simulink model "Model_TranslationEngine64"  (R2022b)
settings: Solver=FixedStepDiscrete  StartTime=0.0  StopTime=5  RelTol=1e-3  EnableMultiTasking=on
InitFcn:
  | % Initialize model
  | ModelSettings=BTConfig.GetModelSettings();
  | 
  | ModelSettings.Validate();
  | 
  | ModelInit;
  | 
  | 
  | % load library data
  | GainLibrary_data;
  | % Load saved values from partition process
  | CapturedConstMask.LoadMapFromFile(bdroot)
StartFcn:
  | % make sure all the simulated RTC requests are found
  | %RTC_SIM_OBJ.ValidateREQs();
undefined symbols (not defined in the file or in its folder): AA, BPLP, Column, NumHFRefBPF, NumHFRefLPF, NumMusicChannels, Row, VolumeMuteConfig
libraries: TuneVar x925, TOP x490, FeaturePath x111, CapturedConstLib x52
(part 27 of 34)

== system Model_TranslationEngine64/ModelPreAmp/DecRate/AudioPilot35/Audiopilot_3_5/NoiseEstimationVariant/RegularNoiseEstimation/HFNoiseEstimatorCoh/PostProcessing/HfImpulseRejection/MinSearch ==
  FlatnessHighIndex : Subsystem  mask(Talaria Trivial Tune TOP){TriggerInit=[-155 320 120 350], TopName=FlatnessHighIndex, TuneName=FlatnessHighIndex, DataTypeOut=single, MaskValue=Config.ImpRejFlatnessHighIndex, TunabilityNumber=1, MinValue=[], MaxValue=[], BankNumber=0, PreOverlay=false, PostOverlay=false, UseSameName=on}
      mask prompts: TriggerInit "Hidden: MoveFcn redraw"; TopName "Name:"; TuneName "Name of TuneVar:"; DataTypeOut "Data type:"; MaskValue "Default Value:"; TunabilityNumber "Tunability:"; MinValue "Min Value:"; MaxValue "Max Value:"; BankNumber "Target memory bank number:"; PreOverlay "Requires pre-overlay action:"; PostOverlay "Requires post-overlay action:"; UseSameName "Use same name for tune variable and TOP"
      mask help: The TuneTOP block encapsultes a Target Overlay Parameter, a Tune Variable, and a Trivial Translation between them.
      mask init:
      | [ok,activeTopPath,activeTunePath] = TuneTOP_Mask.Init(gcbh);
      settings: MoveFcn=TuneTOP_Mask.CB_TriggerInit(gcbh);
      mask Callback TriggerInit: TuneTOP_Mask.CB_TriggerInit(gcbh);
      mask TypeOptions TopName: TOP/TopName
      mask TypeOptions TuneName: Tune Variable/TuneName
      mask TypeOptions DataTypeOut: TOP/DataTypeOut
      mask TypeOptions MaskValue: Tune Variable/MaskValue
      mask TypeOptions TunabilityNumber: Tune Variable/TunabilityNumber
      mask Callback TunabilityNumber: TuneVarMask.CB_TunabilityNumber(gcbh);
      mask TypeOptions MinValue: Tune Variable/MinValue
      mask TypeOptions MaxValue: Tune Variable/MaxValue
      mask TypeOptions BankNumber: TOP/BankNumber
      mask TypeOptions PreOverlay: TOP/PreOverlay
      mask TypeOptions PostOverlay: TOP/PostOverlay
      mask Callback UseSameName: TuneTOP_Mask.CB_UseSameName(gcbh);
      mask DialogControl toolPanel Prompt: Tuning Tool Hints
      mask DialogControl DescriptionGroup Prompt: Description
      mask DialogControl EditDescription Prompt: Edit Description
      mask DialogControl EditDescription Callback: TuneTOP_Mask.CB_EditDescription(gcbh);
      mask DialogControl TunabilityText Prompt: Easy: Changes nearly every tuning.
      mask DialogControl AdvancedPanel Prompt: Advanced
      mask DialogControl ConvertToFullTranslation Prompt: Irreversible conversion to full translation
      mask DialogControl ConvertToFullTranslation Callback: TuneTOP_Mask.CB_ConvertToFullTranslation(gcbh);
      mask DialogControl ErrorContainer Prompt: Error Messages
      mask Display:
      | % retrieve icon definition
      | [path,w,h] = TuneTOP_Mask.Icon();
      | 
      | % retrieve the block's pixel size
      | pos = get(gcbh,'position');
      | bw = pos(3) - pos(1);
      | bh = pos(4) - pos(2);
      | 
      | % draw centered icon
      | xAdj = bw/2 - w/2 + 5;
      | yAdj = bh/2 - h/2 + 4;
      | for i=1:length(path)
      | 	patch(path(i).x+xAdj, path(i).y+yAdj, path(i).rgb);
      | end
      | 
      | % show the top name or an X
      | if (exist('ok','var') && ok)
      | 	text(bw*0.5, bh*0.2, activeTopPath, 'horizontalAlignment', 'center');
      | 	patch(0,0,[1 1 1]);
      | 	patch(bw,bh,[1 1 1]);
      | else
      | 	tx=bw*0.03;
      | 	ty=bh*0.03;
      | 	patch([0 tx bw bw-tx], [ty 0 bh-ty bh], [1 0 0]);
      | 	patch([0 bw-tx bw tx], [bh-ty 0 ty bh], [1 0 0]);
      | end
  FlatnessLowIndex : Subsystem  mask(Talaria Trivial Tune TOP){TriggerInit=[-155 265 120 295], TopName=FlatnessLowIndex, TuneName=FlatnessLowIndex, DataTypeOut=single, MaskValue=Config.ImpRejFlatnessLowIndex, TunabilityNumber=1, MinValue=[], MaxValue=[], BankNumber=0, PreOverlay=false, PostOverlay=false, UseSameName=on}
      mask prompts: TriggerInit "Hidden: MoveFcn redraw"; TopName "Name:"; TuneName "Name of TuneVar:"; DataTypeOut "Data type:"; MaskValue "Default Value:"; TunabilityNumber "Tunability:"; MinValue "Min Value:"; MaxValue "Max Value:"; BankNumber "Target memory bank number:"; PreOverlay "Requires pre-overlay action:"; PostOverlay "Requires post-overlay action:"; UseSameName "Use same name for tune variable and TOP"
      mask help: The TuneTOP block encapsultes a Target Overlay Parameter, a Tune Variable, and a Trivial Translation between them.
      mask init:
      | [ok,activeTopPath,activeTunePath] = TuneTOP_Mask.Init(gcbh);
      settings: MoveFcn=TuneTOP_Mask.CB_TriggerInit(gcbh);
      mask Callback TriggerInit: TuneTOP_Mask.CB_TriggerInit(gcbh);
      mask TypeOptions TopName: TOP/TopName
      mask TypeOptions TuneName: Tune Variable/TuneName
      mask TypeOptions DataTypeOut: TOP/DataTypeOut
      mask TypeOptions MaskValue: Tune Variable/MaskValue
      mask TypeOptions TunabilityNumber: Tune Variable/TunabilityNumber
      mask Callback TunabilityNumber: TuneVarMask.CB_TunabilityNumber(gcbh);
      mask TypeOptions MinValue: Tune Variable/MinValue
      mask TypeOptions MaxValue: Tune Variable/MaxValue
      mask TypeOptions BankNumber: TOP/BankNumber
      mask TypeOptions PreOverlay: TOP/PreOverlay
      mask TypeOptions PostOverlay: TOP/PostOverlay
      mask Callback UseSameName: TuneTOP_Mask.CB_UseSameName(gcbh);
      mask DialogControl toolPanel Prompt: Tuning Tool Hints
      mask DialogControl DescriptionGroup Prompt: Description
      mask DialogControl EditDescription Prompt: Edit Description
      mask DialogControl EditDescription Callback: TuneTOP_Mask.CB_EditDescription(gcbh);
      mask DialogControl TunabilityText Prompt: Easy: Changes nearly every tuning.
      mask DialogControl AdvancedPanel Prompt: Advanced
      mask DialogControl ConvertToFullTranslation Prompt: Irreversible conversion to full translation
      mask DialogControl ConvertToFullTranslation Callback: TuneTOP_Mask.CB_ConvertToFullTranslation(gcbh);
      mask DialogControl ErrorContainer Prompt: Error Messages
      mask Display:
      | % retrieve icon definition
      | [path,w,h] = TuneTOP_Mask.Icon();
      | 
      | % retrieve the block's pixel size
      | pos = get(gcbh,'position');
      | bw = pos(3) - pos(1);
      | bh = pos(4) - pos(2);
      | 
      | % draw centered icon
      | xAdj = bw/2 - w/2 + 5;
      | yAdj = bh/2 - h/2 + 4;
      | for i=1:length(path)
      | 	patch(path(i).x+xAdj, path(i).y+yAdj, path(i).rgb);
      | end
      | 
      | % show the top name or an X
      | if (exist('ok','var') && ok)
      | 	text(bw*0.5, bh*0.2, activeTopPath, 'horizontalAlignment', 'center');
      | 	patch(0,0,[1 1 1]);
      | 	patch(bw,bh,[1 1 1]);
      | else
      | 	tx=bw*0.03;
      | 	ty=bh*0.03;
      | 	patch([0 tx bw bw-tx], [ty 0 bh-ty bh], [1 0 0]);
      | 	patch([0 bw-tx bw tx], [bh-ty 0 ty bh], [1 0 0]);
      | end
  FlatnessThreshold : Subsystem  mask(Talaria Trivial Tune TOP){TriggerInit=[-155 100 120 130], TopName=FlatnessThresh, TuneName=FlatnessThresh, DataTypeOut=single, MaskValue=Config.ImpRejFlatnessThreshold, TunabilityNumber=1, MinValue=[], MaxValue=[], BankNumber=0, PreOverlay=false, PostOverlay=false, UseSameName=on}
      mask prompts: TriggerInit "Hidden: MoveFcn redraw"; TopName "Name:"; TuneName "Name of TuneVar:"; DataTypeOut "Data type:"; MaskValue "Default Value:"; TunabilityNumber "Tunability:"; MinValue "Min Value:"; MaxValue "Max Value:"; BankNumber "Target memory bank number:"; PreOverlay "Requires pre-overlay action:"; PostOverlay "Requires post-overlay action:"; UseSameName "Use same name for tune variable and TOP"
      mask help: The TuneTOP block encapsultes a Target Overlay Parameter, a Tune Variable, and a Trivial Translation between them.
      mask init:
      | [ok,activeTopPath,activeTunePath] = TuneTOP_Mask.Init(gcbh);
      settings: MoveFcn=TuneTOP_Mask.CB_TriggerInit(gcbh);
      mask Callback TriggerInit: TuneTOP_Mask.CB_TriggerInit(gcbh);
      mask TypeOptions TopName: TOP/TopName
      mask TypeOptions TuneName: Tune Variable/TuneName
      mask TypeOptions DataTypeOut: TOP/DataTypeOut
      mask TypeOptions MaskValue: Tune Variable/MaskValue
      mask TypeOptions TunabilityNumber: Tune Variable/TunabilityNumber
      mask Callback TunabilityNumber: TuneVarMask.CB_TunabilityNumber(gcbh);
      mask TypeOptions MinValue: Tune Variable/MinValue
      mask TypeOptions MaxValue: Tune Variable/MaxValue
      mask TypeOptions BankNumber: TOP/BankNumber
      mask TypeOptions PreOverlay: TOP/PreOverlay
      mask TypeOptions PostOverlay: TOP/PostOverlay
      mask Callback UseSameName: TuneTOP_Mask.CB_UseSameName(gcbh);
      mask DialogControl toolPanel Prompt: Tuning Tool Hints
      mask DialogControl DescriptionGroup Prompt: Description
      mask DialogControl EditDescription Prompt: Edit Description
      mask DialogControl EditDescription Callback: TuneTOP_Mask.CB_EditDescription(gcbh);
      mask DialogControl TunabilityText Prompt: Easy: Changes nearly every tuning.
      mask DialogControl AdvancedPanel Prompt: Advanced
      mask DialogControl ConvertToFullTranslation Prompt: Irreversible conversion to full translation
      mask DialogControl ConvertToFullTranslation Callback: TuneTOP_Mask.CB_ConvertToFullTranslation(gcbh);
      mask DialogControl ErrorContainer Prompt: Error Messages
      mask Display:
      | % retrieve icon definition
      | [path,w,h] = TuneTOP_Mask.Icon();
      | 
      | % retrieve the block's pixel size
      | pos = get(gcbh,'position');
      | bw = pos(3) - pos(1);
      | bh = pos(4) - pos(2);
      | 
      | % draw centered icon
      | xAdj = bw/2 - w/2 + 5;
      | yAdj = bh/2 - h/2 + 4;
      | for i=1:length(path)
      | 	patch(path(i).x+xAdj, path(i).y+yAdj, path(i).rgb);
      | end
      | 
      | % show the top name or an X
      | if (exist('ok','var') && ok)
      | 	text(bw*0.5, bh*0.2, activeTopPath, 'horizontalAlignment', 'center');
      | 	patch(0,0,[1 1 1]);
      | 	patch(bw,bh,[1 1 1]);
      | else
      | 	tx=bw*0.03;
      | 	ty=bh*0.03;
      | 	patch([0 tx bw bw-tx], [ty 0 bh-ty bh], [1 0 0]);
      | 	patch([0 bw-tx bw tx], [bh-ty 0 ty bh], [1 0 0]);
      | end
  MinSearchCoef : Subsystem  mask(Talaria Trivial Tune TOP){TriggerInit=[-155 155 120 185], TopName=MinSearchCoef, TuneName=MinSearchCoef, DataTypeOut=single, MaskValue=Config.ImpRejMinSearchCoef, TunabilityNumber=1, MinValue=[], MaxValue=[], BankNumber=0, PreOverlay=false, PostOverlay=false, UseSameName=on}
      mask prompts: TriggerInit "Hidden: MoveFcn redraw"; TopName "Name:"; TuneName "Name of TuneVar:"; DataTypeOut "Data type:"; MaskValue "Default Value:"; TunabilityNumber "Tunability:"; MinValue "Min Value:"; MaxValue "Max Value:"; BankNumber "Target memory bank number:"; PreOverlay "Requires pre-overlay action:"; PostOverlay "Requires post-overlay action:"; UseSameName "Use same name for tune variable and TOP"
      mask help: The TuneTOP block encapsultes a Target Overlay Parameter, a Tune Variable, and a Trivial Translation between them.
      mask init:
      | [ok,activeTopPath,activeTunePath] = TuneTOP_Mask.Init(gcbh);
      settings: MoveFcn=TuneTOP_Mask.CB_TriggerInit(gcbh);
      mask Callback TriggerInit: TuneTOP_Mask.CB_TriggerInit(gcbh);
      mask TypeOptions TopName: TOP/TopName
      mask TypeOptions TuneName: Tune Variable/TuneName
      mask TypeOptions DataTypeOut: TOP/DataTypeOut
      mask TypeOptions MaskValue: Tune Variable/MaskValue
      mask TypeOptions TunabilityNumber: Tune Variable/TunabilityNumber
      mask Callback TunabilityNumber: TuneVarMask.CB_TunabilityNumber(gcbh);
      mask TypeOptions MinValue: Tune Variable/MinValue
      mask TypeOptions MaxValue: Tune Variable/MaxValue
      mask TypeOptions BankNumber: TOP/BankNumber
      mask TypeOptions PreOverlay: TOP/PreOverlay
      mask TypeOptions PostOverlay: TOP/PostOverlay
      mask Callback UseSameName: TuneTOP_Mask.CB_UseSameName(gcbh);
      mask DialogControl toolPanel Prompt: Tuning Tool Hints
      mask DialogControl DescriptionGroup Prompt: Description
      mask DialogControl EditDescription Prompt: Edit Description
      mask DialogControl EditDescription Callback: TuneTOP_Mask.CB_EditDescription(gcbh);
      mask DialogControl TunabilityText Prompt: Easy: Changes nearly every tuning.
      mask DialogControl AdvancedPanel Prompt: Advanced
      mask DialogControl ConvertToFullTranslation Prompt: Irreversible conversion to full translation
      mask DialogControl ConvertToFullTranslation Callback: TuneTOP_Mask.CB_ConvertToFullTranslation(gcbh);
      mask DialogControl ErrorContainer Prompt: Error Messages
      mask Display:
      | % retrieve icon definition
      | [path,w,h] = TuneTOP_Mask.Icon();
      | 
      | % retrieve the block's pixel size
      | pos = get(gcbh,'position');
      | bw = pos(3) - pos(1);
      | bh = pos(4) - pos(2);
      | 
      | % draw centered icon
      | xAdj = bw/2 - w/2 + 5;
      | yAdj = bh/2 - h/2 + 4;
      | for i=1:length(path)
      | 	patch(path(i).x+xAdj, path(i).y+yAdj, path(i).rgb);
      | end
      | 
      | % show the top name or an X
      | if (exist('ok','var') && ok)
      | 	text(bw*0.5, bh*0.2, activeTopPath, 'horizontalAlignment', 'center');
      | 	patch(0,0,[1 1 1]);
      | 	patch(bw,bh,[1 1 1]);
      | else
      | 	tx=bw*0.03;
      | 	ty=bh*0.03;
      | 	patch([0 tx bw bw-tx], [ty 0 bh-ty bh], [1 0 0]);
      | 	patch([0 bw-tx bw tx], [bh-ty 0 ty bh], [1 0 0]);
      | end
  MinSearchMinGain : Subsystem  mask(Talaria Trivial Tune TOP){TriggerInit=[-155 210 120 240], TopName=MinSearchMinGain, TuneName=MinSearchMinGain, DataTypeOut=single, MaskValue=Config.ImpRejMinSearchMinGain, TunabilityNumber=1, MinValue=[], MaxValue=[], BankNumber=0, PreOverlay=false, PostOverlay=false, UseSameName=on}
      mask prompts: TriggerInit "Hidden: MoveFcn redraw"; TopName "Name:"; TuneName "Name of TuneVar:"; DataTypeOut "Data type:"; MaskValue "Default Value:"; TunabilityNumber "Tunability:"; MinValue "Min Value:"; MaxValue "Max Value:"; BankNumber "Target memory bank number:"; PreOverlay "Requires pre-overlay action:"; PostOverlay "Requires post-overlay action:"; UseSameName "Use same name for tune variable and TOP"
      mask help: The TuneTOP block encapsultes a Target Overlay Parameter, a Tune Variable, and a Trivial Translation between them.
      mask init:
      | [ok,activeTopPath,activeTunePath] = TuneTOP_Mask.Init(gcbh);
      settings: MoveFcn=TuneTOP_Mask.CB_TriggerInit(gcbh);
      mask Callback TriggerInit: TuneTOP_Mask.CB_TriggerInit(gcbh);
      mask TypeOptions TopName: TOP/TopName
      mask TypeOptions TuneName: Tune Variable/TuneName
      mask TypeOptions DataTypeOut: TOP/DataTypeOut
      mask TypeOptions MaskValue: Tune Variable/MaskValue
      mask TypeOptions TunabilityNumber: Tune Variable/TunabilityNumber
      mask Callback TunabilityNumber: TuneVarMask.CB_TunabilityNumber(gcbh);
      mask TypeOptions MinValue: Tune Variable/MinValue
      mask TypeOptions MaxValue: Tune Variable/MaxValue
      mask TypeOptions BankNumber: TOP/BankNumber
      mask TypeOptions PreOverlay: TOP/PreOverlay
      mask TypeOptions PostOverlay: TOP/PostOverlay
      mask Callback UseSameName: TuneTOP_Mask.CB_UseSameName(gcbh);
      mask DialogControl toolPanel Prompt: Tuning Tool Hints
      mask DialogControl DescriptionGroup Prompt: Description
      mask DialogControl EditDescription Prompt: Edit Description
      mask DialogControl EditDescription Callback: TuneTOP_Mask.CB_EditDescription(gcbh);
      mask DialogControl TunabilityText Prompt: Easy: Changes nearly every tuning.
      mask DialogControl AdvancedPanel Prompt: Advanced
      mask DialogControl ConvertToFullTranslation Prompt: Irreversible conversion to full translation
      mask DialogControl ConvertToFullTranslation Callback: TuneTOP_Mask.CB_ConvertToFullTranslation(gcbh);
      mask DialogControl ErrorContainer Prompt: Error Messages
      mask Display:
      | % retrieve icon definition
      | [path,w,h] = TuneTOP_Mask.Icon();
      | 
      | % retrieve the block's pixel size
      | pos = get(gcbh,'position');
      | bw = pos(3) - pos(1);
      | bh = pos(4) - pos(2);
      | 
      | % draw centered icon
      | xAdj = bw/2 - w/2 + 5;
      | yAdj = bh/2 - h/2 + 4;
      | for i=1:length(path)
      | 	patch(path(i).x+xAdj, path(i).y+yAdj, path(i).rgb);
      | end
      | 
      | % show the top name or an X
      | if (exist('ok','var') && ok)
      | 	text(bw*0.5, bh*0.2, activeTopPath, 'horizontalAlignment', 'center');
      | 	patch(0,0,[1 1 1]);
      | 	patch(bw,bh,[1 1 1]);
      | else
      | 	tx=bw*0.03;
      | 	ty=bh*0.03;
      | 	patch([0 tx bw bw-tx], [ty 0 bh-ty bh], [1 0 0]);
      | 	patch([0 bw-tx bw tx], [bh-ty 0 ty bh], [1 0 0]);
      | end
  SubWinLen : Subsystem

== system Model_TranslationEngine64/ModelPreAmp/DecRate/AudioPilot35/Audiopilot_3_5/NoiseEstimationVariant/RegularNoiseEstimation/HFNoiseEstimatorCoh/PostProcessing/HfImpulseRejection/SmoothingNoiseFloor ==
  LevelUpdateCoef : Subsystem  mask(Talaria Trivial Tune TOP){TriggerInit=[20 280 265 310], TopName=LevelUpdateCoef, TuneName=LevelUpdateCoef, DataTypeOut=single, MaskValue=Config.ImpRejLevelUpdateCoef, TunabilityNumber=1, MinValue=[], MaxValue=[], BankNumber=0, PreOverlay=false, PostOverlay=false, UseSameName=on}
      mask prompts: TriggerInit "Hidden: MoveFcn redraw"; TopName "Name:"; TuneName "Name of TuneVar:"; DataTypeOut "Data type:"; MaskValue "Default Value:"; TunabilityNumber "Tunability:"; MinValue "Min Value:"; MaxValue "Max Value:"; BankNumber "Target memory bank number:"; PreOverlay "Requires pre-overlay action:"; PostOverlay "Requires post-overlay action:"; UseSameName "Use same name for tune variable and TOP"
      mask help: The TuneTOP block encapsultes a Target Overlay Parameter, a Tune Variable, and a Trivial Translation between them.
      mask init:
      | [ok,activeTopPath,activeTunePath] = TuneTOP_Mask.Init(gcbh);
      settings: MoveFcn=TuneTOP_Mask.CB_TriggerInit(gcbh);
      mask Callback TriggerInit: TuneTOP_Mask.CB_TriggerInit(gcbh);
      mask TypeOptions TopName: TOP/TopName
      mask TypeOptions TuneName: Tune Variable/TuneName
      mask TypeOptions DataTypeOut: TOP/DataTypeOut
      mask TypeOptions MaskValue: Tune Variable/MaskValue
      mask TypeOptions TunabilityNumber: Tune Variable/TunabilityNumber
      mask Callback TunabilityNumber: TuneVarMask.CB_TunabilityNumber(gcbh);
      mask TypeOptions MinValue: Tune Variable/MinValue
      mask TypeOptions MaxValue: Tune Variable/MaxValue
      mask TypeOptions BankNumber: TOP/BankNumber
      mask TypeOptions PreOverlay: TOP/PreOverlay
      mask TypeOptions PostOverlay: TOP/PostOverlay
      mask Callback UseSameName: TuneTOP_Mask.CB_UseSameName(gcbh);
      mask DialogControl toolPanel Prompt: Tuning Tool Hints
      mask DialogControl DescriptionGroup Prompt: Description
      mask DialogControl EditDescription Prompt: Edit Description
      mask DialogControl EditDescription Callback: TuneTOP_Mask.CB_EditDescription(gcbh);
      mask DialogControl TunabilityText Prompt: Easy: Changes nearly every tuning.
      mask DialogControl AdvancedPanel Prompt: Advanced
      mask DialogControl ConvertToFullTranslation Prompt: Irreversible conversion to full translation
      mask DialogControl ConvertToFullTranslation Callback: TuneTOP_Mask.CB_ConvertToFullTranslation(gcbh);
      mask DialogControl ErrorContainer Prompt: Error Messages
      mask Display:
      | % retrieve icon definition
      | [path,w,h] = TuneTOP_Mask.Icon();
      | 
      | % retrieve the block's pixel size
      | pos = get(gcbh,'position');
      | bw = pos(3) - pos(1);
      | bh = pos(4) - pos(2);
      | 
      | % draw centered icon
      | xAdj = bw/2 - w/2 + 5;
      | yAdj = bh/2 - h/2 + 4;
      | for i=1:length(path)
      | 	patch(path(i).x+xAdj, path(i).y+yAdj, path(i).rgb);
      | end
      | 
      | % show the top name or an X
      | if (exist('ok','var') && ok)
      | 	text(bw*0.5, bh*0.2, activeTopPath, 'horizontalAlignment', 'center');
      | 	patch(0,0,[1 1 1]);
      | 	patch(bw,bh,[1 1 1]);
      | else
      | 	tx=bw*0.03;
      | 	ty=bh*0.03;
      | 	patch([0 tx bw bw-tx], [ty 0 bh-ty bh], [1 0 0]);
      | 	patch([0 bw-tx bw tx], [bh-ty 0 ty bh], [1 0 0]);
      | end

== system Model_TranslationEngine64/ModelPreAmp/DecRate/AudioPilot35/Audiopilot_3_5/NoiseEstimationVariant/RegularNoiseEstimation/HFNoiseEstimatorCoh/PostProcessing/HfSlew/attack ==
  TOP : TOP/TOP  TriggerInit=[200 107 420 153]  TopName=AttackDbPerSample  DataTypeOut=single  BankNumber=0  PreOverlay=false  PostOverlay=false  Role=Automatic
      settings: SourceProductName=Bose Talaria
  TranslateTrigger : TuneVar/TranslateTrigger  TriggerInit=[81 5 119 60]
      settings: SourceProductName=Bose Talaria
  Tune Variable : TuneVar/TuneVar  TuneName=AttackDbPerS  SpecifyMaxSize=off  VariableDim=1 (Row)  MaxSize=[1 1]  TunabilityNumber=1  MinValue=[]  MaxValue=[]  TriggerInit=[-300 105 -100 155]  MaskValue=Config.SlewAttackDbpersec
      settings: SourceProductName=Bose Talaria
  sec2sample : MATLAB Function  TreatAsAtomicUnit=on
  wires:
  sec2sample/1(y) -> TOP/1
  Tune Variable/1 -> sec2sample/1(u)  "AttackDbPerS"
  TranslateTrigger/1 -> sec2sample/Trigger

== system Model_TranslationEngine64/ModelPreAmp/DecRate/AudioPilot35/Audiopilot_3_5/NoiseEstimationVariant/RegularNoiseEstimation/HFNoiseEstimatorCoh/PostProcessing/HfSlew/decay ==
  TOP : TOP/TOP  TriggerInit=[200 110 395 150]  TopName=DecayDbPerSample  DataTypeOut=single  BankNumber=0  PreOverlay=false  PostOverlay=false  Role=Automatic
      settings: SourceProductName=Bose Talaria
  TranslateTrigger : TuneVar/TranslateTrigger  TriggerInit=[81 5 119 60]
      settings: SourceProductName=Bose Talaria
  Tune Variable : TuneVar/TuneVar  TuneName=DecayDbPerS  SpecifyMaxSize=off  VariableDim=1 (Row)  MaxSize=[1 1]  TunabilityNumber=1  MinValue=[]  MaxValue=[]  TriggerInit=[-300 110 -65 150]  MaskValue=Config.SlewDecayDbpersec
      settings: SourceProductName=Bose Talaria
  sec2sample : MATLAB Function  TreatAsAtomicUnit=on
  wires:
  TranslateTrigger/1 -> sec2sample/Trigger
  Tune Variable/1 -> sec2sample/1(u)  "DecayDbPerS"
  sec2sample/1(y) -> TOP/1

== system Model_TranslationEngine64/ModelPreAmp/DecRate/AudioPilot35/Audiopilot_3_5/NoiseEstimationVariant/RegularNoiseEstimation/HFNoiseEstimatorCoh/PostProcessing/HfSlew/threshold ==
  TOP : TOP/TOP  TriggerInit=[440 20 585 80]  TopName=ThresholdDb  DataTypeOut=single  BankNumber=BankNumber  PreOverlay=PreOverlay  PostOverlay=PostOverlay  Role=Automatic
      settings: SourceProductName=Bose Talaria
  TrivialTranslation : TuneVar/TrivialTranslation  TriggerInit=[300 28 350 72]
      settings: SourceProductName=Bose Talaria
  Tune Variable : TuneVar/TuneVar  TuneName=ThresholdDb  SpecifyMaxSize=off  VariableDim=1 (Row)  MaxSize=[1 1]  TunabilityNumber=1  MinValue=MinValue  MaxValue=MaxValue  TriggerInit=[20 25 190 75]  MaskValue=MaskValue
      settings: SourceProductName=Bose Talaria
  wires:
  TrivialTranslation/1 -> TOP/1
  Tune Variable/1 -> TrivialTranslation/1  "ThresholdDb"

== system Model_TranslationEngine64/ModelPreAmp/DecRate/AudioPilot35/Audiopilot_3_5/NoiseEstimationVariant/RegularNoiseEstimation/HFNoiseEstimatorCoh/PreProcessing/Anti-Aliasing Filter/InnerLink ==
  PoolIirTunableWithReset : Subsystem  mask(Bose Pool IIR Tunable){FeatureName=PreprocessAntiAlias, Config=Config}
      mask prompts: FeatureName "Filter name/purpose"; Config "PoolIirTunableWithResetConfig"
      mask help:
      | Pool IIR Tunable is a configurable multi-channel IIR filter that supports one or more channels. This block offers flexibility of tuning the number of stages and coefficients. Different filter coefficients and number of stages (biquads) can be used for each channel filter. The Pool IIR Tunable block supports different implementations, which could be configured at build-time:
      |
      | (i)   Generic: IIR filter code not optimized for any processor
      | (ii)  SharcCore: IIR filters executing on core (uses pooliir.asm CRL)
      | (iii) SharcGulAccel: IIR filters executing on IIR hardware accelerator, offloading MIPS usage from core
      | (iv) SharcGxpAccel: IIR filters take advantage of additional accelerators available on GXP processor
      | (v)  Hexagon: TBD
      |
      | NOTE: When using Pool IIR for Sharc-plus based processors, the codeWorkMemory buffer and input buffer should always be mapped to L1 memory to optimize MIPS utilization and avoid audio artifacts.
      |
      | For more information, please see 'Help'.
      mask init:
      | blkh=gcbh;
      | Config=BTConfig.Assert(blkh,Config);
      | 
      | BTConfig.InitSetFeatureIfPresent(blkh,'FeatureName');
      | Config.Validate();
      | Config.DoMaskInit(blkh);
      mask Help:
      | <b>Input signals: </b>
      | AudioIn: input channels [frame size x number of channels]
      | ResetTrigger: trigger to reset internal state buffer (usually preferred as a post RMDL step)
      | 
      | <b>Output signals: </b>
      | AudioOut: output channels [frame size x number of channels]
      | 
      | <b>Mask parameters: </b>
      | PoolIirTunableWithResetConfig
      | Filter name/purpose
      mask TypeOptions FeatureName: FeaturePath/FeatureName
      mask Callback Config: BTConfig.CallbackHideIfPresent(gcbh,{'FeatureName'});
      mask Display: DrawPoolIirIcon;

== system Model_TranslationEngine64/ModelPreAmp/DecRate/AudioPilot35/Audiopilot_3_5/NoiseEstimationVariant/RegularNoiseEstimation/HFNoiseEstimatorCoh/PreProcessing/Bandpass or Lowpass Filter/InnerLink ==
  PoolIirTunableWithReset : Subsystem  mask(Bose Pool IIR Tunable){FeatureName=PreprocessBandpassLowpass, Config=Config}
      mask prompts: FeatureName "Filter name/purpose"; Config "PoolIirTunableWithResetConfig"
      mask help:
      | Pool IIR Tunable is a configurable multi-channel IIR filter that supports one or more channels. This block offers flexibility of tuning the number of stages and coefficients. Different filter coefficients and number of stages (biquads) can be used for each channel filter. The Pool IIR Tunable block supports different implementations, which could be configured at build-time:
      |
      | (i)   Generic: IIR filter code not optimized for any processor
      | (ii)  SharcCore: IIR filters executing on core (uses pooliir.asm CRL)
      | (iii) SharcGulAccel: IIR filters executing on IIR hardware accelerator, offloading MIPS usage from core
      | (iv) SharcGxpAccel: IIR filters take advantage of additional accelerators available on GXP processor
      | (v)  Hexagon: TBD
      |
      | NOTE: When using Pool IIR for Sharc-plus based processors, the codeWorkMemory buffer and input buffer should always be mapped to L1 memory to optimize MIPS utilization and avoid audio artifacts.
      |
      | For more information, please see 'Help'.
      mask init:
      | blkh=gcbh;
      | Config=BTConfig.Assert(blkh,Config);
      | 
      | BTConfig.InitSetFeatureIfPresent(blkh,'FeatureName');
      | Config.Validate();
      | Config.DoMaskInit(blkh);
      mask Help:
      | <b>Input signals: </b>
      | AudioIn: input channels [frame size x number of channels]
      | ResetTrigger: trigger to reset internal state buffer (usually preferred as a post RMDL step)
      | 
      | <b>Output signals: </b>
      | AudioOut: output channels [frame size x number of channels]
      | 
      | <b>Mask parameters: </b>
      | PoolIirTunableWithResetConfig
      | Filter name/purpose
      mask TypeOptions FeatureName: FeaturePath/FeatureName
      mask Callback Config: BTConfig.CallbackHideIfPresent(gcbh,{'FeatureName'});
      mask Display: DrawPoolIirIcon;

== system Model_TranslationEngine64/ModelPreAmp/DecRate/AudioPilot35/Audiopilot_3_5/NoiseEstimationVariant/RegularNoiseEstimation/LFNoiseEstimatorCoh/LfPreProcess/FilterMic/InnerLink ==
  PoolIirTunableWithReset : Subsystem  mask(Bose Pool IIR Tunable){FeatureName=Mic, Config=Config}
      mask prompts: FeatureName "Filter name/purpose"; Config "PoolIirTunableWithResetConfig"
      mask help:
      | Pool IIR Tunable is a configurable multi-channel IIR filter that supports one or more channels. This block offers flexibility of tuning the number of stages and coefficients. Different filter coefficients and number of stages (biquads) can be used for each channel filter. The Pool IIR Tunable block supports different implementations, which could be configured at build-time:
      |
      | (i)   Generic: IIR filter code not optimized for any processor
      | (ii)  SharcCore: IIR filters executing on core (uses pooliir.asm CRL)
      | (iii) SharcGulAccel: IIR filters executing on IIR hardware accelerator, offloading MIPS usage from core
      | (iv) SharcGxpAccel: IIR filters take advantage of additional accelerators available on GXP processor
      | (v)  Hexagon: TBD
      |
      | NOTE: When using Pool IIR for Sharc-plus based processors, the codeWorkMemory buffer and input buffer should always be mapped to L1 memory to optimize MIPS utilization and avoid audio artifacts.
      |
      | For more information, please see 'Help'.
      mask init:
      | blkh=gcbh;
      | Config=BTConfig.Assert(blkh,Config);
      | 
      | BTConfig.InitSetFeatureIfPresent(blkh,'FeatureName');
      | Config.Validate();
      | Config.DoMaskInit(blkh);
      mask Help:
      | <b>Input signals: </b>
      | AudioIn: input channels [frame size x number of channels]
      | ResetTrigger: trigger to reset internal state buffer (usually preferred as a post RMDL step)
      | 
      | <b>Output signals: </b>
      | AudioOut: output channels [frame size x number of channels]
      | 
      | <b>Mask parameters: </b>
      | PoolIirTunableWithResetConfig
      | Filter name/purpose
      mask TypeOptions FeatureName: FeaturePath/FeatureName
      mask Callback Config: BTConfig.CallbackHideIfPresent(gcbh,{'FeatureName'});
      mask Display: DrawPoolIirIcon;

== system Model_TranslationEngine64/ModelPreAmp/DecRate/AudioPilot35/Audiopilot_3_5/NoiseEstimationVariant/RegularNoiseEstimation/LFNoiseEstimatorCoh/LfPreProcess/FilterRef/InnerLink ==
  PoolIirTunableWithReset : Subsystem  mask(Bose Pool IIR Tunable){FeatureName=Ref, Config=Config}
      mask prompts: FeatureName "Filter name/purpose"; Config "PoolIirTunableWithResetConfig"
      mask help:
      | Pool IIR Tunable is a configurable multi-channel IIR filter that supports one or more channels. This block offers flexibility of tuning the number of stages and coefficients. Different filter coefficients and number of stages (biquads) can be used for each channel filter. The Pool IIR Tunable block supports different implementations, which could be configured at build-time:
      |
      | (i)   Generic: IIR filter code not optimized for any processor
      | (ii)  SharcCore: IIR filters executing on core (uses pooliir.asm CRL)
      | (iii) SharcGulAccel: IIR filters executing on IIR hardware accelerator, offloading MIPS usage from core
      | (iv) SharcGxpAccel: IIR filters take advantage of additional accelerators available on GXP processor
      | (v)  Hexagon: TBD
      |
      | NOTE: When using Pool IIR for Sharc-plus based processors, the codeWorkMemory buffer and input buffer should always be mapped to L1 memory to optimize MIPS utilization and avoid audio artifacts.
      |
      | For more information, please see 'Help'.
      mask init:
      | blkh=gcbh;
      | Config=BTConfig.Assert(blkh,Config);
      | 
      | BTConfig.InitSetFeatureIfPresent(blkh,'FeatureName');
      | Config.Validate();
      | Config.DoMaskInit(blkh);
      mask Help:
      | <b>Input signals: </b>
      | AudioIn: input channels [frame size x number of channels]
      | ResetTrigger: trigger to reset internal state buffer (usually preferred as a post RMDL step)
      | 
      | <b>Output signals: </b>
      | AudioOut: output channels [frame size x number of channels]
      | 
      | <b>Mask parameters: </b>
      | PoolIirTunableWithResetConfig
      | Filter name/purpose
      mask TypeOptions FeatureName: FeaturePath/FeatureName
      mask Callback Config: BTConfig.CallbackHideIfPresent(gcbh,{'FeatureName'});
      mask Display: DrawPoolIirIcon;

== system Model_TranslationEngine64/ModelPreAmp/DecRate/AudioPilot35/Audiopilot_3_5/NoiseEstimationVariant/RegularNoiseEstimation/LFNoiseEstimatorCoh/SpeedBoundsAndNoiseSlew/LfNoiseSlew/Attack ==
  TOP : TOP/TOP  TriggerInit=[125 85 330 145]  TopName=AttackDbPerSample  DataTypeOut=single  BankNumber=0  PreOverlay=false  PostOverlay=false  Role=Automatic
      settings: SourceProductName=Bose Talaria
  TranslateTrigger : TuneVar/TranslateTrigger  TriggerInit=[-19 -10 19 45]
      settings: SourceProductName=Bose Talaria
  Tune Variable : TuneVar/TuneVar  TuneName=AttackDbPerS  SpecifyMaxSize=off  VariableDim=1 (Row)  MaxSize=[1 1]  TunabilityNumber=1  MinValue=[]  MaxValue=[]  TriggerInit=[-385 90 -215 140]  MaskValue=Config.SlewAttackDbpersec
      settings: SourceProductName=Bose Talaria
  sec2sample : MATLAB Function  TreatAsAtomicUnit=on
  wires:
  sec2sample/1(y) -> TOP/1
  Tune Variable/1 -> sec2sample/1(u)  "AttackDbPerS"
  TranslateTrigger/1 -> sec2sample/Trigger

== system Model_TranslationEngine64/ModelPreAmp/DecRate/AudioPilot35/Audiopilot_3_5/NoiseEstimationVariant/RegularNoiseEstimation/LFNoiseEstimatorCoh/SpeedBoundsAndNoiseSlew/LfNoiseSlew/Decay ==
  TOP : TOP/TOP  TriggerInit=[100 85 315 145]  TopName=DecayDbPerSample  DataTypeOut=single  BankNumber=0  PreOverlay=false  PostOverlay=false  Role=Automatic
      settings: SourceProductName=Bose Talaria
  TranslateTrigger : TuneVar/TranslateTrigger  TriggerInit=[-19 -10 19 45]
      settings: SourceProductName=Bose Talaria
  Tune Variable : TuneVar/TuneVar  TuneName=DecayDbPerS  SpecifyMaxSize=off  VariableDim=1 (Row)  MaxSize=[1 1]  TunabilityNumber=1  MinValue=[]  MaxValue=[]  TriggerInit=[-385 90 -215 140]  MaskValue=Config.SlewDecayDbpersec
      settings: SourceProductName=Bose Talaria
  sec2sample : MATLAB Function  TreatAsAtomicUnit=on
  wires:
  TranslateTrigger/1 -> sec2sample/Trigger
  Tune Variable/1 -> sec2sample/1(u)  "DecayDbPerS"
  sec2sample/1(y) -> TOP/1

== system Model_TranslationEngine64/ModelPreAmp/DecRate/AudioPilot35/Audiopilot_3_5/NoiseEstimationVariant/RegularNoiseEstimation/LFNoiseEstimatorCoh/SpeedBoundsAndNoiseSlew/LfNoiseSlew/SlowSlew ==
  TOP : TOP/TOP  TriggerInit=[100 87 320 143]  TopName=SlowDbPerSample  DataTypeOut=single  BankNumber=0  PreOverlay=false  PostOverlay=false  Role=Automatic
      settings: SourceProductName=Bose Talaria
  TranslateTrigger : TuneVar/TranslateTrigger  TriggerInit=[-19 -10 19 45]
      settings: SourceProductName=Bose Talaria
  Tune Variable : TuneVar/TuneVar  TuneName=SlowDbPerS  SpecifyMaxSize=off  VariableDim=1 (Row)  MaxSize=[1 1]  TunabilityNumber=1  MinValue=[]  MaxValue=[]  TriggerInit=[-335 90 -165 140]  MaskValue=Config.SlewSlowSlewDbpersec
      settings: SourceProductName=Bose Talaria
  sec2sample : MATLAB Function  TreatAsAtomicUnit=on
  wires:
  sec2sample/1(y) -> TOP/1
  Tune Variable/1 -> sec2sample/1(u)  "SlowDbPerS"
  TranslateTrigger/1 -> sec2sample/Trigger

== system Model_TranslationEngine64/ModelPreAmp/DecRate/AudioPilot35/Audiopilot_3_5/NoiseEstimationVariant/RegularNoiseEstimation/LFNoiseEstimatorCoh/SpeedBoundsAndNoiseSlew/LfNoiseSlew/Threshold ==
  TOP : TOP/TOP  TriggerInit=[440 20 585 80]  TopName=ThresholdDb  DataTypeOut=single  BankNumber=BankNumber  PreOverlay=PreOverlay  PostOverlay=PostOverlay  Role=Automatic
      settings: SourceProductName=Bose Talaria
  TrivialTranslation : TuneVar/TrivialTranslation  TriggerInit=[300 28 350 72]
      settings: SourceProductName=Bose Talaria
  Tune Variable : TuneVar/TuneVar  TuneName=ThresholdDb  SpecifyMaxSize=off  VariableDim=1 (Row)  MaxSize=[1 1]  TunabilityNumber=1  MinValue=MinValue  MaxValue=MaxValue  TriggerInit=[20 25 190 75]  MaskValue=MaskValue
      settings: SourceProductName=Bose Talaria
  wires:
  TrivialTranslation/1 -> TOP/1
  Tune Variable/1 -> TrivialTranslation/1  "ThresholdDb"

== system Model_TranslationEngine64/ModelPreAmp/DecRate/AudioPilot35/Audiopilot_3_5/NoiseEstimationVariant/RegularNoiseEstimation/LFNoiseEstimatorCoh/SpeedBoundsAndNoiseSlew/SpeedBounds/axis ==
  TOP : TOP/TOP  TriggerInit=[440 20 585 80]  TopName=Axis  DataTypeOut=single  BankNumber=BankNumber  PreOverlay=PreOverlay  PostOverlay=PostOverlay  Role=Automatic
      settings: SourceProductName=Bose Talaria
  TrivialTranslation : TuneVar/TrivialTranslation  TriggerInit=[300 28 350 72]
      settings: SourceProductName=Bose Talaria
  Tune Variable : TuneVar/TuneVar  TuneName=Axis  SpecifyMaxSize=off  VariableDim=1 (Row)  MaxSize=[1 1]  TunabilityNumber=1  MinValue=MinValue  MaxValue=MaxValue  TriggerInit=[20 25 190 75]  MaskValue=MaskValue
      settings: SourceProductName=Bose Talaria
  wires:
  TrivialTranslation/1 -> TOP/1
  Tune Variable/1 -> TrivialTranslation/1  "Axis"

== system Model_TranslationEngine64/ModelPreAmp/DecRate/AudioPilot35/Audiopilot_3_5/NoiseEstimationVariant/RegularNoiseEstimation/LFNoiseEstimatorCoh/SpeedBoundsAndNoiseSlew/SpeedBounds/max ==
  TOP : TOP/TOP  TriggerInit=[440 20 585 80]  TopName=MaxDbspl  DataTypeOut=single  BankNumber=BankNumber  PreOverlay=PreOverlay  PostOverlay=PostOverlay  Role=Automatic
      settings: SourceProductName=Bose Talaria
  TrivialTranslation : TuneVar/TrivialTranslation  TriggerInit=[300 28 350 72]
      settings: SourceProductName=Bose Talaria
  Tune Variable : TuneVar/TuneVar  TuneName=MaxDbspl  SpecifyMaxSize=off  VariableDim=1 (Row)  MaxSize=[1 1]  TunabilityNumber=1  MinValue=MinValue  MaxValue=MaxValue  TriggerInit=[20 25 190 75]  MaskValue=MaskValue
      settings: SourceProductName=Bose Talaria
  wires:
  TrivialTranslation/1 -> TOP/1
  Tune Variable/1 -> TrivialTranslation/1  "MaxDbspl"

== system Model_TranslationEngine64/ModelPreAmp/DecRate/AudioPilot35/Audiopilot_3_5/NoiseEstimationVariant/RegularNoiseEstimation/LFNoiseEstimatorCoh/SpeedBoundsAndNoiseSlew/SpeedBounds/min ==
  TOP : TOP/TOP  TriggerInit=[440 -15 585 45]  TopName=MinDbspl  DataTypeOut=single  BankNumber=0  PreOverlay=false  PostOverlay=false  Role=Automatic
      settings: SourceProductName=Bose Talaria
  TOP1 : TOP/TOP  TriggerInit=[440 55 585 115]  TopName=MinBoundsLowestValDbspl  DataTypeOut=single  BankNumber=0  PreOverlay=false  PostOverlay=false  Role=Automatic
      settings: SourceProductName=Bose Talaria
  TranslateTrigger : TuneVar/TranslateTrigger  TriggerInit=[306 -100 344 -45]
      settings: SourceProductName=Bose Talaria
  Trivial Translation : MATLAB Function  TreatAsAtomicUnit=on
  Tune Variable : TuneVar/TuneVar  TuneName=MindBSPL  SpecifyMaxSize=off  VariableDim=1 (Row)  MaxSize=[1 1]  TunabilityNumber=1  MinValue=[]  MaxValue=[]  TriggerInit=[20 25 190 75]  MaskValue=Config.SpeedBoundsMindBSPL
      settings: SourceProductName=Bose Talaria
  wires:
  Tune Variable/1 -> Trivial Translation/1(Tune1)  "MindBSPL"
  Trivial Translation/1(TOP) -> TOP/1
  TranslateTrigger/1 -> Trivial Translation/Trigger
  Trivial Translation/2(minBoundsLowestVal) -> TOP1/1

== system Model_TranslationEngine64/ModelPreAmp/DecRate/AudioPilot35/Audiopilot_3_5/NoiseEstimationVariant/RegularNoiseEstimation/LFNoiseEstimatorCoh/SpeedBoundsAndNoiseSlew/SpeedBounds/on ==
  TOP : TOP/TOP  TriggerInit=[440 20 585 80]  TopName=On  DataTypeOut=single  BankNumber=BankNumber  PreOverlay=PreOverlay  PostOverlay=PostOverlay  Role=Automatic
      settings: SourceProductName=Bose Talaria
  TrivialTranslation : TuneVar/TrivialTranslation  TriggerInit=[300 28 350 72]
      settings: SourceProductName=Bose Talaria
  Tune Variable : TuneVar/TuneVar  TuneName=On  SpecifyMaxSize=off  VariableDim=1 (Row)  MaxSize=[1 1]  TunabilityNumber=1  MinValue=MinValue  MaxValue=MaxValue  TriggerInit=[20 25 190 75]  MaskValue=MaskValue
      settings: SourceProductName=Bose Talaria
  wires:
  TrivialTranslation/1 -> TOP/1
  Tune Variable/1 -> TrivialTranslation/1  "On"

== system Model_TranslationEngine64/ModelPreAmp/DecRate/Medusa5H1/MedusaHoligram/Medusa5H1 Part 2/Decimated-Rate FDP/Fdp/FreqDomainProcessing/CalculateAndApplyCoefficients/DeciRate ==
  Calculate coefficients : Subsystem
      settings: LibrarySourceBlock=MedusaFdp/MedusaDeciRateFdp/DeciRateFdp/FreqDomainProcessing/Calculate coefficients

== system Model_TranslationEngine64/ModelPreAmp/DecRate/Medusa5H1/MedusaHoligram/Medusa5H1 Part 2/Decimated-Rate FDP/Fdp/FreqDomainProcessing/CalculateAndApplyCoefficients/FullRate ==

== system Model_TranslationEngine64/ModelPreAmp/DecRate/Medusa5H1/MedusaHoligram/Medusa5H1 Part 2/Full-Rate FDP/Fdp/FreqDomainProcessing/CalculateAndApplyCoefficients/DeciRate ==

== system Model_TranslationEngine64/ModelPreAmp/DecRate/Medusa5H1/MedusaHoligram/Medusa5H1 Part 2/Full-Rate FDP/Fdp/FreqDomainProcessing/CalculateAndApplyCoefficients/FullRate ==
  Calculate coefficients : Subsystem

== system Model_TranslationEngine64/ModelPreAmp/DecRate/Medusa5H1/MedusaHoligram/Medusa5H1 Part 3/On/Expand Tail Components/Tail Component EQ/InnerLink/PoolIirTunableWithReset ==
  CapturedTuneConst : CapturedConstLib/CapturedConst  TriggerInit=[-600 302 -500 338]  Role=Automatic
      settings: SourceProductName=Bose Talaria
  FeaturePath : FeaturePath/FeaturePath  FeatureName=tailCompEQ  IsGroup=off  GroupNumber=-1  IsModule=off  TriggerInit=[-750 -81 -635 26]
      settings: SourceProductName=Bose Talaria
  TOP : TOP/TOP  TriggerInit=[-145 187 5 243]  TopName=PooliirNumStages  DataTypeOut=uint32  BankNumber=0  PreOverlay=false  PostOverlay=Config.VariantObj.PostOverlayRequired  Role=Automatic
      settings: SourceProductName=Bose Talaria
  TOP1 : TOP/TOP  TriggerInit=[-140 277 10 333]  TopName=pooliirCoeffs  DataTypeOut=single  BankNumber=0  PreOverlay=false  PostOverlay=Config.VariantObj.PostOverlayRequired  Role=Automatic
      settings: SourceProductName=Bose Talaria
  TranslateTrigger : TuneVar/TranslateTrigger  TriggerInit=[-339 35 -301 90]
      settings: SourceProductName=Bose Talaria
  Translation : MATLAB Function  TreatAsAtomicUnit=on  mask{MaxNumStages=Config.MaxNumStages, VariantUint8=Config.Variant.Uint8Str}
      mask prompts: VariantUint8 "Variant"
  Tune Variable1 : TuneVar/TuneVar  TuneName=numStages  SpecifyMaxSize=off  VariableDim=1 (Row)  MaxSize=[1 1]  TunabilityNumber=1  MinValue=[]  MaxValue=[]  TriggerInit=[-750 235 -580 285]  MaskValue=Config.TuneDefaults.NumStages
      settings: SourceProductName=Bose Talaria
  Tune Variable2 : TuneVar/TuneVar  TuneName=sosCoefficients  SpecifyMaxSize=on  VariableDim=1 (Row)  MaxSize=[Config.MaxNumStages 6]  TunabilityNumber=1  MinValue=[]  MaxValue=[]  TriggerInit=[-750 175 -580 225]  MaskValue=Config.TuneDefaults.SosCoefficients
      settings: SourceProductName=Bose Talaria
  wires:
  CapturedTuneConst/1 -> Translation/3(NumChannels)
  Tune Variable1/1 -> Translation/2(NumStages)  "numStages"
  Translation/1(PoolNumStages) -> TOP/1
  Translation/2(PoolCoeffs) -> TOP1/1
  Tune Variable2/1 -> Translation/1(RawSOS)  "sosCoefficients"
  TranslateTrigger/1 -> Translation/Trigger

== system Model_TranslationEngine64/ModelPreAmp/DecRate/Medusa5H1/MedusaHoligram/Medusa5H1 Part 3/On/Full-rate Mixer/Full-Rate Mixer with CAE & Fade Ramper/Fade Tuning/Backward Downmix Max ==
  TOP : TOP/TOP  TriggerInit=[440 20 585 80]  TopName=BackwardDownmixMax  DataTypeOut=single  BankNumber=0  PreOverlay=false  PostOverlay=false  Role=Automatic
      settings: SourceProductName=Bose Talaria
  TranslateTrigger : TuneVar/TranslateTrigger  TriggerInit=[286 -100 324 -45]
      settings: SourceProductName=Bose Talaria
  Trivial Translation : MATLAB Function  TreatAsAtomicUnit=on
  Tune Variable : TuneVar/TuneVar  TuneName=BackwardDownmixMax  SpecifyMaxSize=off  VariableDim=1 (Row)  MaxSize=[1 1]  TunabilityNumber=1  MinValue=[0]  MaxValue=[1]  TriggerInit=[-65 25 105 75]  MaskValue=MedusaFRMTune.BackwardDownmixMax
      settings: SourceProductName=Bose Talaria
  wires:
  Tune Variable/1 -> Trivial Translation/1(BackwardDownmixMax)  "BackwardDownmixMax"
  Trivial Translation/1(TOP) -> TOP/1
  TranslateTrigger/1 -> Trivial Translation/Trigger

== system Model_TranslationEngine64/ModelPreAmp/DecRate/Medusa5H1/MedusaHoligram/Medusa5H1 Part 3/On/Full-rate Mixer/Full-Rate Mixer with CAE & Fade Ramper/Fade Tuning/Backward Downmix Threshold ==
  TOP : TOP/TOP  TriggerInit=[440 20 585 80]  TopName=BackwardDownmixThreshold  DataTypeOut=single  BankNumber=0  PreOverlay=false  PostOverlay=false  Role=Automatic
      settings: SourceProductName=Bose Talaria
  TranslateTrigger : TuneVar/TranslateTrigger  TriggerInit=[306 -100 344 -45]
      settings: SourceProductName=Bose Talaria
  Trivial Translation : MATLAB Function  TreatAsAtomicUnit=on
  Tune Variable : TuneVar/TuneVar  TuneName=BackwardDownmixThreshold  SpecifyMaxSize=off  VariableDim=1 (Row)  MaxSize=[1 1]  TunabilityNumber=1  MinValue=[0]  MaxValue=[1]  TriggerInit=[-75 25 95 75]  MaskValue=MedusaFRMTune.BackwardDownmixThreshold
      settings: SourceProductName=Bose Talaria
  wires:
  Tune Variable/1 -> Trivial Translation/1(BackwardDownmixThreshold)  "BackwardDownmixThreshold"
  Trivial Translation/1(TOP) -> TOP/1
  TranslateTrigger/1 -> Trivial Translation/Trigger

== system Model_TranslationEngine64/ModelPreAmp/DecRate/Medusa5H1/MedusaHoligram/Medusa5H1 Part 3/On/Full-rate Mixer/Full-Rate Mixer with CAE & Fade Ramper/Fade Tuning/Downmix Weights CS ==
  TOP : TOP/TOP  TriggerInit=[440 -15 600 45]  TopName=DownmixWeights_CS  DataTypeOut=single  BankNumber=0  PreOverlay=false  PostOverlay=false  Role=Automatic
      settings: SourceProductName=Bose Talaria
  TOP1 : TOP/TOP  TriggerInit=[440 55 600 115]  TopName=DownmixWeights_CS_CAE  DataTypeOut=single  BankNumber=0  PreOverlay=false  PostOverlay=false  Role=Automatic
      settings: SourceProductName=Bose Talaria
  TranslateTrigger : TuneVar/TranslateTrigger  TriggerInit=[256 -100 294 -45]
      settings: SourceProductName=Bose Talaria
  Trivial Translation : MATLAB Function  TreatAsAtomicUnit=on
  Tune Variable : TuneVar/TuneVar  TuneName=DownmixWeights_CS  SpecifyMaxSize=off  VariableDim=1 (Row)  MaxSize=[1 1]  TunabilityNumber=1  MinValue=[0]  MaxValue=[1]  TriggerInit=[-85 25 85 75]  MaskValue=MedusaFRMTune.downmix_wts_CS
      settings: SourceProductName=Bose Talaria
  wires:
  Tune Variable/1 -> Trivial Translation/1(downmix_wts_CS)  "DownmixWeights_CS"
  Trivial Translation/1(TOP) -> TOP/1
  TranslateTrigger/1 -> Trivial Translation/Trigger
  Trivial Translation/2(TOP_CAE) -> TOP1/1

== system Model_TranslationEngine64/ModelPreAmp/DecRate/Medusa5H1/MedusaHoligram/Medusa5H1 Part 3/On/Full-rate Mixer/Full-Rate Mixer with CAE & Fade Ramper/Fade Tuning/Downmix Weights Left ==
  TOP : TOP/TOP  TriggerInit=[440 -15 605 45]  TopName=DownmixWeights_Left  DataTypeOut=single  BankNumber=0  PreOverlay=false  PostOverlay=false  Role=Automatic
      settings: SourceProductName=Bose Talaria
  TOP1 : TOP/TOP  TriggerInit=[440 55 605 115]  TopName=DownmixWeights_Left_CAE  DataTypeOut=single  BankNumber=0  PreOverlay=false  PostOverlay=false  Role=Automatic
      settings: SourceProductName=Bose Talaria
  TranslateTrigger : TuneVar/TranslateTrigger  TriggerInit=[266 -100 304 -45]
      settings: SourceProductName=Bose Talaria
  Trivial Translation : MATLAB Function  TreatAsAtomicUnit=on
  Tune Variable : TuneVar/TuneVar  TuneName=DownmixWeights_Left  SpecifyMaxSize=off  VariableDim=1 (Row)  MaxSize=[1 1]  TunabilityNumber=1  MinValue=[0]  MaxValue=[1]  TriggerInit=[-80 25 90 75]  MaskValue=MedusaFRMTune.downmix_wts_Left
      settings: SourceProductName=Bose Talaria
  wires:
  Tune Variable/1 -> Trivial Translation/1(downmix_wts_Left)  "DownmixWeights_Left"
  Trivial Translation/1(TOP) -> TOP/1
  TranslateTrigger/1 -> Trivial Translation/Trigger
  Trivial Translation/2(TOP_CAE) -> TOP1/1

== system Model_TranslationEngine64/ModelPreAmp/DecRate/Medusa5H1/MedusaHoligram/Medusa5H1 Part 3/On/Full-rate Mixer/Full-Rate Mixer with CAE & Fade Ramper/Fade Tuning/Downmix Weights Right ==
  TOP : TOP/TOP  TriggerInit=[475 -15 645 45]  TopName=DownmixWeights_Right  DataTypeOut=single  BankNumber=0  PreOverlay=false  PostOverlay=false  Role=Automatic
      settings: SourceProductName=Bose Talaria
  TOP1 : TOP/TOP  TriggerInit=[475 55 645 115]  TopName=DownmixWeights_Right_CAE  DataTypeOut=single  BankNumber=0  PreOverlay=false  PostOverlay=false  Role=Automatic
      settings: SourceProductName=Bose Talaria
  TranslateTrigger : TuneVar/TranslateTrigger  TriggerInit=[306 -100 344 -45]
      settings: SourceProductName=Bose Talaria
  Trivial Translation : MATLAB Function  TreatAsAtomicUnit=on
  Tune Variable : TuneVar/TuneVar  TuneName=DownmixWeights_Right  SpecifyMaxSize=off  VariableDim=1 (Row)  MaxSize=[1 1]  TunabilityNumber=1  MinValue=[0]  MaxValue=[1]  TriggerInit=[-40 25 130 75]  MaskValue=MedusaFRMTune.downmix_wts_Right
      settings: SourceProductName=Bose Talaria
  wires:
  Tune Variable/1 -> Trivial Translation/1(downmix_wts_Right)  "DownmixWeights_Right"
  Trivial Translation/1(TOP) -> TOP/1
  TranslateTrigger/1 -> Trivial Translation/Trigger
  Trivial Translation/2(TOP_CAE) -> TOP1/1
